simulink model "V511_L4_TDI"  (R2020b)
settings: Solver=VariableStepAuto  StartTime=0.0  StopTime=110  MaxStep=0.01  RelTol=1e-3
settings Model: Creator=td  LastModifiedBy=Maxim
settings DataIOCC: ReturnWorkspaceOutputs=off
settings DebuggingCC: ArithmeticOperatorsInVariantConditions=warning
settings SFSimCC: CustomCodeUndefinedFunction=UseInterfaceOnly

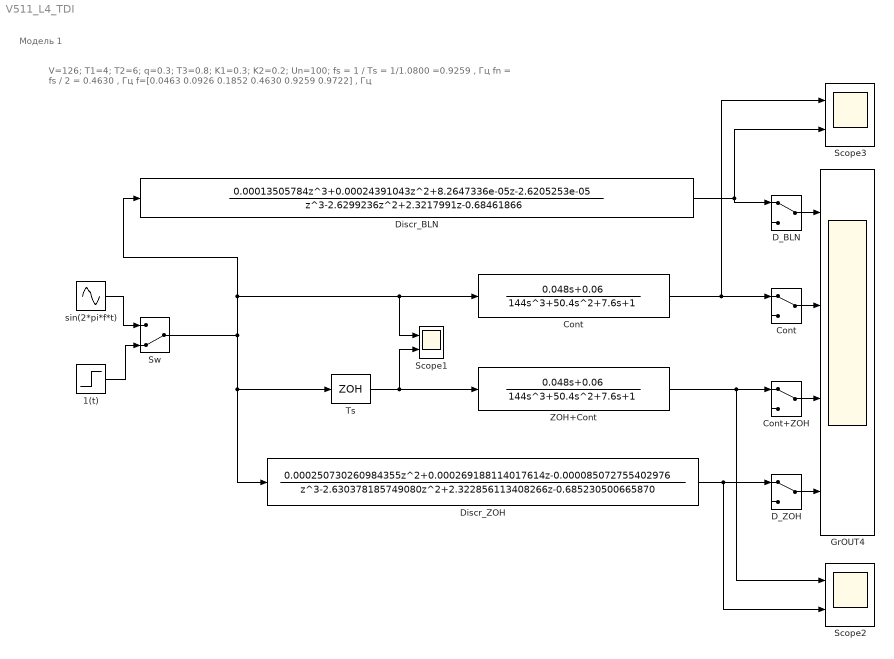
== system V511_L4_TDI ==
  note: Модель 1
  note: V=126; T1=4; T2=6; q=0.3; T3=0.8; K1=0.3; K2=0.2; Un=100;
      |
      | fs = 1 / Ts = 1/1.0800 =0.9259 , Гц
      | fn = fs / 2 = 0.4630 , Гц
      |
      | f=[0.0463 0.0926 0.1852 0.4630 0.9259 0.9722] , Гц
  " Sw  " : ManualSwitch  CurrentSetting=0
  1(t) : Step  Time=0  SampleTime=0
  Cont : TransferFcn  Numerator=[0.048 0.06]  Denominator=[144 50.4 7.6 1]
  "Cont " : ManualSwitch
  "Cont+ZOH " : ManualSwitch
  D_BLN : ManualSwitch
  D_ZOH : ManualSwitch
  Discr_BLN : DiscreteTransferFcn  Numerator="[ 0.00013505784  0.00024391043  8.2647336e-05 -2.6205253e-05 ]"  Denominator="[ 1     -2.6299236      2.3217991    -0.68461866 ]"  SampleTime=1.08
  Discr_ZOH : DiscreteTransferFcn  Numerator="[0   0.000250730260984355   0.000269188114017614  -0.000085072755402976]"  Denominator="[1  -2.630378185749080   2.322856113408266  -0.685230500665870]"  SampleTime=1.08
  GrOUT4 : Scope  NumInputPorts=4
  Scope1 : Scope  NumInputPorts=2
  Scope2 : Scope  NumInputPorts=2
  Scope3 : Scope  NumInputPorts=2
  Ts : ZeroOrderHold  SampleTime=0.54
  ZOH+Cont : TransferFcn  Numerator=[0.048 0.06]  Denominator=[144 50.4 7.6 1]
  sin(2*pi*f*t) : Sin  Frequency=2*pi*0.9759  SampleTime=0
  wires:
  " Sw  "/1 -> Discr_BLN/1, Cont/1, Scope1/1, Discr_ZOH/1, Ts/1
  Ts/1 -> ZOH+Cont/1, Scope1/2
  Cont/1 -> "Cont "/1, Scope3/1
  Discr_BLN/1 -> D_BLN/1, Scope3/2
  Discr_ZOH/1 -> Scope2/2, D_ZOH/1
  ZOH+Cont/1 -> Scope2/1, "Cont+ZOH "/1
  D_BLN/1 -> GrOUT4/1
  "Cont "/1 -> GrOUT4/2
  "Cont+ZOH "/1 -> GrOUT4/3
  D_ZOH/1 -> GrOUT4/4
  sin(2*pi*f*t)/1 -> " Sw  "/1
  1(t)/1 -> " Sw  "/2
